simulink model "Assignement_Simulink"  (R2022b)
settings: Solver=ode8  StartTime=0.0  StopTime=50000  FixedStep=0.1  RelTol=1e-3
values from neighbouring files (symbols this model uses):
  a = 16371e3    (= 16371000)    [Assignement_Script.m]
  A0 = eye(3,3)    [Assignement_Script.m]
  A1 = 0.02    [Assignement_Script.m]
  A2 = A1    (= 0.02)    [Assignement_Script.m]
  A3 = A1    (= 0.02)    [Assignement_Script.m]
  alpha_1 = 0.5    [Assignement_Script.m]
  alpha_2 = 0.5    [Assignement_Script.m]
  C_d = 2.1    [Assignement_Script.m]
  e = 0    [Assignement_Script.m]
  epsilon = 0.4093    [Assignement_Script.m]
  G = 6.6743e-11    [Assignement_Script.m]
  H0 = sqrt(g_10^2+g_11^2+h_11^2)    [Assignement_Script.m]
  i = 0.1    [Assignement_Script.m]
  I = 12/23.342 *diag([0.343,0.344,0.286])    [Assignement_Script.m]
  j_B = [0.01;0.05;0.01]    [Assignement_Script.m]
  k_d_detumbling = 0.12    [Assignement_Script.m]
  k_d_nadir = 0.12    [Assignement_Script.m]
  k_p_nadir = 0.12    [Assignement_Script.m]
  M_Earth = 5.972e24    (= 5.972e+24)    [Assignement_Script.m]
  n = sqrt(G*M_Earth/a^3)    [Assignement_Script.m]
  n_sun = 2*pi/T_sun    (= 1.99238499086e-07)    [Assignement_Script.m]
  omega_detumbling = [0; 0; n_SC]    [Assignement_Script.m]
  omega_nadir = omega_detumbling    [Assignement_Script.m]
  P = F_e/c    (= 4.52666666667e-06)    [Assignement_Script.m]
  position = 1e-2*[15,0,0;0,5,0;-15,0,0;0,-5,0;0,0,10;                                     0,0,-10;0,20,10;0,20,10;0,-20,10;0,-20,10]    [Assignement_Script.m]
  R_Earth = 6.378e6    (= 6378000)    [Assignement_Script.m]
  R_sun = 149597870000    [Assignement_Script.m]
  rhoD_vector = ones(10,1)*0.1    [Assignement_Script.m]
  rhoS_vector = ones(10,1)*0.5    [Assignement_Script.m]
  Surfaces_Matrix = [2e-2;6e-2;2e-2;6e-2;3e-2;3e-2;12e-2;                                                     12e-2;12e-2;12e-2]    [Assignement_Script.m]
  theta0 = 3/2*pi    (= 4.71238898038)    [Assignement_Script.m]
  Theta_m = deg2rad(11.5)    [Assignement_Script.m]
  time_detumbling = 500    [Assignement_Script.m]
  Versor_Surfaces_Matrix = [  1 , 0 ,-1 , 0 , 0 , 0 , 0 , 0 , 0 , 0 ... (first row only)    [Assignement_Script.m]
  w0 = [0;0;0.01]    [Assignement_Script.m]
  w_Earth = 7.2916e-5    (= 7.2916e-05)    [Assignement_Script.m]
undefined symbols (not defined in the file or in its folder): Gyroscope, HS, RW, SunSensor
libraries: simulink_extras x14, vrlib x11, matrix_library x10, sharedutil x10
(part 1 of 2)
settings Model: Creator=ludov  LastModifiedBy=ludov

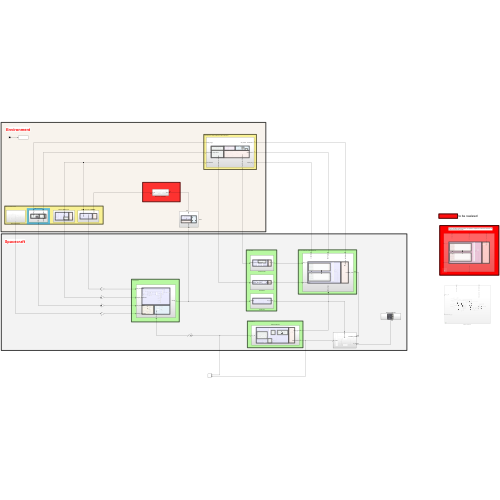
[thumbnail: Simulink's stored preview of the top-level diagram]
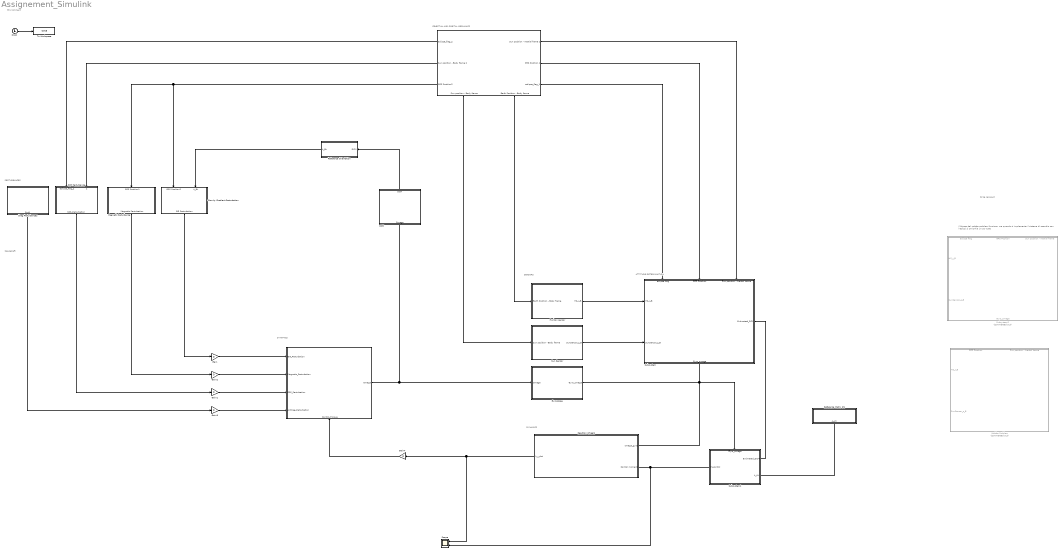
== system Assignement_Simulink ==
  note: il blocco del wabba problem funziona, ma quando si implementa il sistema di scambio con l'eclissi si smicnhia un po' tutto
  note: Environment
  note: ATTITUDE DETERMINATION
  note: to be rewiewd
  note: DYNAMICS
  note: SENSORS
  note: CELESTIAL AND ORBITAL MECHANICS
  note: PERTURBANCES
  note: Spacecraft
  note: DYNAMICS
  " " : Subsystem
      settings: PortSchema="{\"entries\":[{\"content\":{\"sides\":[{\"content\":{\"connectorIds\":[\"Out6\",\"Out7\",\"Out8\"]},\"type\":\"ConnectorPlacement.EquallySpacedRectSide\",\"uuid\":\"e47ba2f2-6418-4f5c-a13b-aa90bdbafa09\"},{\"content\":{\"connectorIds\":[\"Out1\",\"Out2\",\"Out3\"],\"side\":\"RIGHT\"},\"type\":\"ConnectorPlacement.EquallySpacedRectSide\",\"uuid\":\"03bc7c76-661c-4c4e-84cf-6f77fb49d6cb\"},{\"content\":{\"connectorIds\":[],\"side\":\"TOP\"},\"type\":\"ConnectorPlacement.EquallySpacedRectSide\",\"uuid\":\"b7f23859-8b5f-4f36-86dd-1ae14c2fa2a2\"},{\"content\":{\"connectorIds\":[\"Out4\",\"Out5\"],\"side\":\"BOTTOM\"},\"type\":\"ConnectorPlacement.EquallySpacedRectSide\",\"uuid\":\"86089f92-8549-4212-b188-d7aa2d93da25\"}]},\"type\":\"ConnectorPlacement.EquallySpacedConnector\",\"uuid\":\"9d05c9f0-b3f6-416c-9c64-67f4b43926de\"}],\"packageUris\":[\"http://schema.mathworks.com/mf0/Connector/R2020b\"],\"version\":\"1.0\"}"
  "  " : Subsystem
      settings: PortSchema="{\"entries\":[{\"content\":{\"sides\":[{\"content\":{\"connectorIds\":[\"In1\",\"In2\",\"In3\",\"In4\"]},\"type\":\"ConnectorPlacement.EquallySpacedRectSide\",\"uuid\":\"aab80584-571d-4a71-b544-a0aeb6cc6c33\"},{\"content\":{\"connectorIds\":[\"Out1\"],\"side\":\"RIGHT\"},\"type\":\"ConnectorPlacement.EquallySpacedRectSide\",\"uuid\":\"24834e7f-96cf-4bd4-9d1e-2a40a9329077\"},{\"content\":{\"connectorIds\":[],\"side\":\"TOP\"},\"type\":\"ConnectorPlacement.EquallySpacedRectSide\",\"uuid\":\"d2051258-9c4b-4932-9464-9f9a506b88fb\"},{\"content\":{\"connectorIds\":[\"In5\"],\"side\":\"BOTTOM\"},\"type\":\"ConnectorPlacement.EquallySpacedRectSide\",\"uuid\":\"d87f08de-6428-4147-8fa3-4a4fdf5058ef\"}]},\"type\":\"ConnectorPlacement.EquallySpacedConnector\",\"uuid\":\"040bda51-1336-4023-88c4-8bbc78e4cc03\"}],\"packageUris\":[\"http://schema.mathworks.com/mf0/Connector/R2020b\"],\"version\":\"1.0\"}"
  " Magnetic Perturbance " : Subsystem
      settings: PortSchema="{\"entries\":[{\"content\":{\"sides\":[{\"content\":{\"connectorIds\":[]},\"type\":\"ConnectorPlacement.EquallySpacedRectSide\",\"uuid\":\"f02812cb-12c0-4612-9b94-50dc5ff6800f\"},{\"content\":{\"connectorIds\":[],\"side\":\"RIGHT\"},\"type\":\"ConnectorPlacement.EquallySpacedRectSide\",\"uuid\":\"f399267d-7809-425c-9d5e-8a09b98f84d1\"},{\"content\":{\"connectorIds\":[\"In1\"],\"side\":\"TOP\"},\"type\":\"ConnectorPlacement.EquallySpacedRectSide\",\"uuid\":\"723c78fa-3a63-413c-a07c-383f30094b4e\"},{\"content\":{\"connectorIds\":[\"Out1\"],\"side\":\"BOTTOM\"},\"type\":\"ConnectorPlacement.EquallySpacedRectSide\",\"uuid\":\"6e581abe-40d1-4528-bc1e-881c860c6457\"}]},\"type\":\"ConnectorPlacement.EquallySpacedConnector\",\"uuid\":\"57020123-0faa-4eee-b688-9329c8cd004b\"}],\"packageUris\":[\"http://schema.mathworks.com/mf0/Connector/R2020b\"],\"version\":\"1.0\"}"
  " SRP Perturbance" : Subsystem
      settings: PortSchema="{\"entries\":[{\"content\":{\"sides\":[{\"content\":{\"connectorIds\":[]},\"type\":\"ConnectorPlacement.EquallySpacedRectSide\",\"uuid\":\"e985e879-37b8-4f0c-a60b-74d5e4b5102c\"},{\"content\":{\"connectorIds\":[],\"side\":\"RIGHT\"},\"type\":\"ConnectorPlacement.EquallySpacedRectSide\",\"uuid\":\"1f0cb419-685e-4dd3-ab14-45869a41b9c2\"},{\"content\":{\"connectorIds\":[\"In1\",\"In2\"],\"side\":\"TOP\"},\"type\":\"ConnectorPlacement.EquallySpacedRectSide\",\"uuid\":\"f8cfa143-02f3-47d6-960d-90021c53ea82\"},{\"content\":{\"connectorIds\":[\"Out1\"],\"side\":\"BOTTOM\"},\"type\":\"ConnectorPlacement.EquallySpacedRectSide\",\"uuid\":\"2a12fd6d-c4b7-49e6-8cbf-522d896783f6\"}]},\"type\":\"ConnectorPlacement.EquallySpacedConnector\",\"uuid\":\"8752746d-e23a-4760-aab6-3f1c0a06bc69\"}],\"packageUris\":[\"http://schema.mathworks.com/mf0/Connector/R2020b\"],\"version\":\"1.0\"}"
  Clock : Clock
  DCM : Subsystem
      settings: PortSchema="{\"entries\":[{\"content\":{\"sides\":[{\"content\":{\"connectorIds\":[]},\"type\":\"ConnectorPlacement.EquallySpacedRectSide\",\"uuid\":\"36de77ec-8153-48fc-ae5a-ad0b0e2d3ce0\"},{\"content\":{\"connectorIds\":[],\"side\":\"RIGHT\"},\"type\":\"ConnectorPlacement.EquallySpacedRectSide\",\"uuid\":\"5bb36846-76d5-425c-bf3c-97c4283359fa\"},{\"content\":{\"connectorIds\":[\"Out1\"],\"side\":\"TOP\"},\"type\":\"ConnectorPlacement.EquallySpacedRectSide\",\"uuid\":\"8effcbf1-f39c-4e11-8297-2eedf506960c\"},{\"content\":{\"connectorIds\":[\"In1\"],\"side\":\"BOTTOM\"},\"type\":\"ConnectorPlacement.EquallySpacedRectSide\",\"uuid\":\"d53277ca-d1bd-4bb5-ab75-f8d5bccd248f\"}]},\"type\":\"ConnectorPlacement.EquallySpacedConnector\",\"uuid\":\"1130cf8d-ea10-4dfb-b209-46460bb57623\"}],\"packageUris\":[\"http://schema.mathworks.com/mf0/Connector/R2020b\"],\"version\":\"1.0\"}"
  Drag Perturbances : Subsystem
      settings: PortSchema="{\"entries\":[{\"content\":{\"sides\":[{\"content\":{\"connectorIds\":[]},\"type\":\"ConnectorPlacement.EquallySpacedRectSide\",\"uuid\":\"890f3e81-eae3-4d82-b131-a6b55e2e4e7e\"},{\"content\":{\"connectorIds\":[],\"side\":\"RIGHT\"},\"type\":\"ConnectorPlacement.EquallySpacedRectSide\",\"uuid\":\"fd77badb-3975-40f3-b2ef-8bc06b5f839c\"},{\"content\":{\"connectorIds\":[],\"side\":\"TOP\"},\"type\":\"ConnectorPlacement.EquallySpacedRectSide\",\"uuid\":\"74a13749-9f47-4ab9-b559-aa1ff3776051\"},{\"content\":{\"connectorIds\":[\"Out1\"],\"side\":\"BOTTOM\"},\"type\":\"ConnectorPlacement.EquallySpacedRectSide\",\"uuid\":\"ad5dbb3d-b795-4ab1-8885-dcb70df44dd7\"}]},\"type\":\"ConnectorPlacement.EquallySpacedConnector\",\"uuid\":\"adbac40e-e9e4-4933-ac77-075f4cd465ab\"}],\"packageUris\":[\"http://schema.mathworks.com/mf0/Connector/R2020b\"],\"version\":\"1.0\"}"
  Gain{,1..4} (5 alike) : Gain  Gain=0
  Gravity Gradient Perturbation : Subsystem
      settings: PortSchema="{\"entries\":[{\"content\":{\"sides\":[{\"content\":{\"connectorIds\":[]},\"type\":\"ConnectorPlacement.EquallySpacedRectSide\",\"uuid\":\"0f339a99-129b-4972-909e-aa08984290af\"},{\"content\":{\"connectorIds\":[],\"side\":\"RIGHT\"},\"type\":\"ConnectorPlacement.EquallySpacedRectSide\",\"uuid\":\"c349fcfc-19e0-4c37-99ec-428747fba93f\"},{\"content\":{\"connectorIds\":[\"In1\",\"In2\"],\"side\":\"TOP\"},\"type\":\"ConnectorPlacement.EquallySpacedRectSide\",\"uuid\":\"2ac505f4-7a46-421c-9759-99416a32691b\"},{\"content\":{\"connectorIds\":[\"Out1\"],\"side\":\"BOTTOM\"},\"type\":\"ConnectorPlacement.EquallySpacedRectSide\",\"uuid\":\"46063fda-cf86-410f-90fc-74dd4707f3ff\"}]},\"type\":\"ConnectorPlacement.EquallySpacedConnector\",\"uuid\":\"8656328d-f6ad-4baa-a1ea-e4d5445b99d9\"}],\"packageUris\":[\"http://schema.mathworks.com/mf0/Connector/R2020b\"],\"version\":\"1.0\"}"
  Gyroscope : Subsystem
  Horizon sensor : Subsystem
  Reaction Wheels : Subsystem
  Reference Matrix #1 : Subsystem
      settings: PortSchema="{\"entries\":[{\"content\":{\"sides\":[{\"content\":{\"connectorIds\":[]},\"type\":\"ConnectorPlacement.EquallySpacedRectSide\",\"uuid\":\"bcca36cf-8ac8-4df2-8c27-820de1fbb3ba\"},{\"content\":{\"connectorIds\":[],\"side\":\"RIGHT\"},\"type\":\"ConnectorPlacement.EquallySpacedRectSide\",\"uuid\":\"8624ce1f-10a4-46ad-9e5b-1a912f6d00ca\"},{\"content\":{\"connectorIds\":[],\"side\":\"TOP\"},\"type\":\"ConnectorPlacement.EquallySpacedRectSide\",\"uuid\":\"93036ba9-ac54-41ed-8cce-c13b1508dd7a\"},{\"content\":{\"connectorIds\":[\"Out1\"],\"side\":\"BOTTOM\"},\"type\":\"ConnectorPlacement.EquallySpacedRectSide\",\"uuid\":\"73593883-c463-4775-a781-721666040d63\"}]},\"type\":\"ConnectorPlacement.EquallySpacedConnector\",\"uuid\":\"7208a640-a625-4ee7-a86a-82274cfadb5b\"}],\"packageUris\":[\"http://schema.mathworks.com/mf0/Connector/R2020b\"],\"version\":\"1.0\"}"
  Reference Orientation : Subsystem
  Scope : Scope  NumInputPorts=2
  Subsystem : Subsystem
      settings: PortSchema="{\"entries\":[{\"content\":{\"sides\":[{\"content\":{\"connectorIds\":[\"In1\",\"In2\"]},\"type\":\"ConnectorPlacement.EquallySpacedRectSide\",\"uuid\":\"904c8655-8bda-40bc-8851-83b785dfa15e\"},{\"content\":{\"connectorIds\":[\"Out1\"],\"side\":\"RIGHT\"},\"type\":\"ConnectorPlacement.EquallySpacedRectSide\",\"uuid\":\"2c7420fa-7058-46da-8085-0ee08a188acb\"},{\"content\":{\"connectorIds\":[\"In3\",\"In4\",\"In5\"],\"side\":\"TOP\"},\"type\":\"ConnectorPlacement.EquallySpacedRectSide\",\"uuid\":\"499ed007-25d9-4559-b35a-ae71d71143f6\"},{\"content\":{\"connectorIds\":[\"In6\"],\"side\":\"BOTTOM\"},\"type\":\"ConnectorPlacement.EquallySpacedRectSide\",\"uuid\":\"c0208a51-188e-4d0b-a2a2-f21f47979d66\"}]},\"type\":\"ConnectorPlacement.EquallySpacedConnector\",\"uuid\":\"16926250-8c74-4bf5-939a-452d45825930\"}],\"packageUris\":[\"http://schema.mathworks.com/mf0/Connector/R2020b\"],\"version\":\"1.0\"}"
  Subsystem1 : Subsystem
      settings: PortSchema="{\"entries\":[{\"content\":{\"sides\":[{\"content\":{\"connectorIds\":[\"In1\",\"In2\"]},\"type\":\"ConnectorPlacement.EquallySpacedRectSide\",\"uuid\":\"bcca36cf-8ac8-4df2-8c27-820de1fbb3ba\"},{\"content\":{\"connectorIds\":[\"Out1\"],\"side\":\"RIGHT\"},\"type\":\"ConnectorPlacement.EquallySpacedRectSide\",\"uuid\":\"8624ce1f-10a4-46ad-9e5b-1a912f6d00ca\"},{\"content\":{\"connectorIds\":[\"In3\"],\"side\":\"TOP\"},\"type\":\"ConnectorPlacement.EquallySpacedRectSide\",\"uuid\":\"93036ba9-ac54-41ed-8cce-c13b1508dd7a\"}]},\"type\":\"ConnectorPlacement.EquallySpacedConnector\",\"uuid\":\"7208a640-a625-4ee7-a86a-82274cfadb5b\"}],\"packageUris\":[\"http://schema.mathworks.com/mf0/Connector/R2020b\"],\"version\":\"1.0\"}"
  Subsystem2 : Subsystem  Commented=on
      settings: PortSchema="{\"entries\":[{\"content\":{\"sides\":[{\"content\":{\"connectorIds\":[\"In1\",\"In2\"]},\"type\":\"ConnectorPlacement.EquallySpacedRectSide\",\"uuid\":\"904c8655-8bda-40bc-8851-83b785dfa15e\"},{\"content\":{\"connectorIds\":[],\"side\":\"RIGHT\"},\"type\":\"ConnectorPlacement.EquallySpacedRectSide\",\"uuid\":\"2c7420fa-7058-46da-8085-0ee08a188acb\"},{\"content\":{\"connectorIds\":[\"In3\",\"In4\",\"In5\"],\"side\":\"TOP\"},\"type\":\"ConnectorPlacement.EquallySpacedRectSide\",\"uuid\":\"499ed007-25d9-4559-b35a-ae71d71143f6\"},{\"content\":{\"connectorIds\":[\"In6\"],\"side\":\"BOTTOM\"},\"type\":\"ConnectorPlacement.EquallySpacedRectSide\",\"uuid\":\"c0208a51-188e-4d0b-a2a2-f21f47979d66\"}]},\"type\":\"ConnectorPlacement.EquallySpacedConnector\",\"uuid\":\"16926250-8c74-4bf5-939a-452d45825930\"}],\"packageUris\":[\"http://schema.mathworks.com/mf0/Connector/R2020b\"],\"version\":\"1.0\"}"
  Sun Sensor : Subsystem
  To Workspace : ToWorkspace  VariableName=time  SampleTime=-1
  "Wabba Problem   " : Subsystem  Commented=on
      settings: PortSchema="{\"entries\":[{\"content\":{\"sides\":[{\"content\":{\"connectorIds\":[\"In1\",\"In2\"]},\"type\":\"ConnectorPlacement.EquallySpacedRectSide\",\"uuid\":\"692c6d3d-a8f2-499c-91a9-b0c93e98f75e\"},{\"content\":{\"connectorIds\":[],\"side\":\"RIGHT\"},\"type\":\"ConnectorPlacement.EquallySpacedRectSide\",\"uuid\":\"1ce742a3-ce52-440c-800e-89beb75c5b36\"},{\"content\":{\"connectorIds\":[\"In3\",\"In4\"],\"side\":\"TOP\"},\"type\":\"ConnectorPlacement.EquallySpacedRectSide\",\"uuid\":\"136b807f-193f-4c92-b740-36ee5afae013\"},{\"content\":{\"connectorIds\":[],\"side\":\"BOTTOM\"},\"type\":\"ConnectorPlacement.EquallySpacedRectSide\",\"uuid\":\"f63666af-b04e-4ebd-b890-e9da3a257b46\"}]},\"type\":\"ConnectorPlacement.EquallySpacedConnector\",\"uuid\":\"09b5b65f-bc7f-44eb-8e09-c61a35babfb4\"}],\"packageUris\":[\"http://schema.mathworks.com/mf0/Connector/R2020b\"],\"version\":\"1.0\"}"
  wires:
  DCM/1(DCM) -> Reference Orientation/1(DCM)
  "  "/1(Omega) -> DCM/1(Omega), Gyroscope/1(Omega)
  " SRP Perturbance"/1(SRP_Perturbation) -> Gain1/1
  " Magnetic Perturbance "/1(Magnetic Perturbation) -> Gain2/1
  Drag Perturbances/1(Out1) -> Gain3/1
  Reference Orientation/1(A_BL) -> Gravity Gradient Perturbation/2(A_BL)
  Gravity Gradient Perturbation/1(GG Perturbation) -> Gain/1
  " "/5(Earth Position - Body frame) -> Horizon sensor/1(Earth Position - Body frame)
  " "/4(Sun position - Body frame) -> Sun Sensor/1(Sun position - Body frame)
  " "/3(eclipse_flag_1) -> Subsystem/3(eclipse flag)
  " "/1(Sun position - Inertial frame 1) -> Subsystem/5(Sun position - Inertial frame)
  " "/2(GPS Position 1) -> Subsystem/4(GPS Position)
  Gain/1 -> "  "/1(GG_Perturbation)
  Gain1/1 -> "  "/3(SRP_Perturbation)
  Gain2/1 -> "  "/2(Magnetic_Perturbation)
  Gain3/1 -> "  "/4(AirDrag_Perturbation)
  Gyroscope/1(Gyro_omega) -> Reaction Wheels/1(omega_gyro), Subsystem1/3(Gyro_omega), Subsystem/6(Gyro_omega)
  Horizon sensor/1(HS_r_B) -> Subsystem/1(HS_r_B)
  Sun Sensor/1(SunSensor_s_B) -> Subsystem/2(SunSensor_s_B)
  " "/8(GPS Position2) -> " Magnetic Perturbance "/1(GPS Position1), Gravity Gradient Perturbation/1(GPS Position2)
  " "/7(Sun position - Body frame 2) -> " SRP Perturbance"/2(Sun position - Inertial frame 2)
  Reaction Wheels/1(h_r_dot) -> Scope/1, Gain4/1
  Clock/1 -> To Workspace/1
  " "/6(eclipse_flag_2) -> " SRP Perturbance"/1(eclipse_flag_2)
  Subsystem1/1(M_control) -> Scope/2, Reaction Wheels/2(Control moment)
  Gain4/1 -> "  "/5(Control_Torque)
  Reference Matrix #1/1(A_LN) -> Subsystem1/2(A_LN)
  Subsystem/1(Extimated_DCM) -> Subsystem1/1(Extimated_DCM)

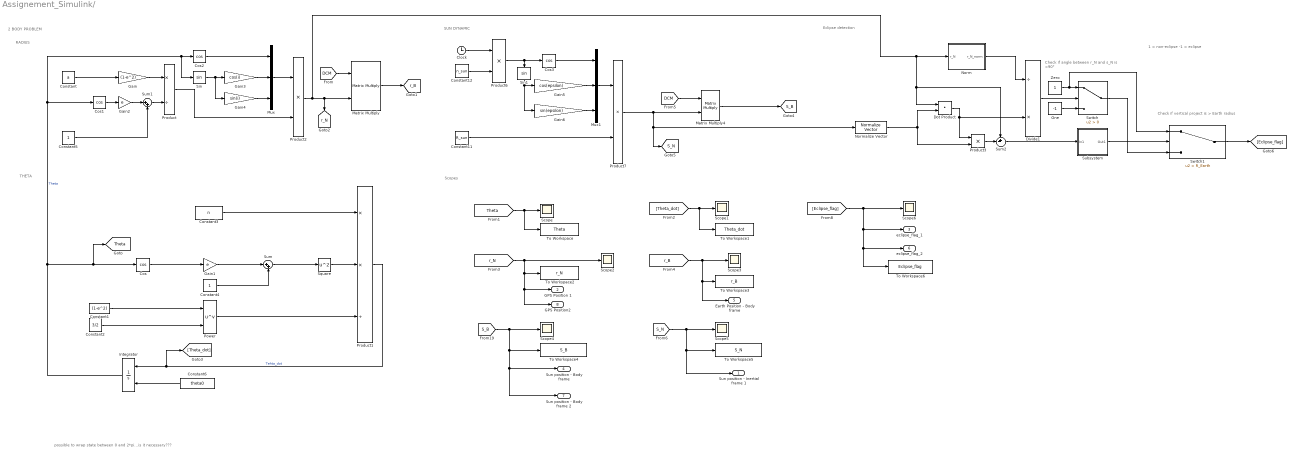
== system Assignement_Simulink/  ==
  note: 1 = non-eclipse
      | -1 = eclipse
  note: Check if vertical project is > Earth
      |  radius
  note: Check if angle between r_N
      |  and s_N is >90°
  note: Eclipse detection
  note: possible to wrap state between 0 and 2*pi...is it necessary???
  note: RADIUS
  note: 2 BODY PROBLEM
  note: THETA
  note: Scopes
  note: SUN DYNAMIC
  Clock : Clock
  Constant : Constant  Value=a
  Constant1 : Constant  Value=(1-e^2)
  Constant11 : Constant  Value=R_sun
  Constant12 : Constant  Value=n_sun
  Constant2 : Constant  Value=3/2
  Constant3 : Constant  Value=n
  Constant4 : Constant
  Constant5 : Constant
  Constant6 : Constant  Value=theta0
  Cos{,1..3} (4 alike) : Trigonometry  Operator=cos
  Divide1 : Product  Inputs=/*
  Dot Product : DotProduct  OutDataTypeStr=Inherit: Inherit via internal rule
  Gain : Gain  Gain=(1-e^2)
  Gain1 : Gain  Gain=e
  Gain2 : Gain  Gain=e
  Gain3 : Gain  Gain=cos(i)
  Gain4 : Gain  Gain=sin(i)
  Gain5 : Gain  Gain=cos(epsilon)
  Gain6 : Gain  Gain=sin(epsilon)
  Integrator : Integrator  InitialConditionSource=external  WrappedStateUpperValue=2*pi  WrappedStateLowerValue=0
  Matrix Multiply : Product  Multiplication=Matrix(*)
  Matrix Multiply4 : Product  Multiplication=Matrix(*)
  Mux : Mux  Inputs=3
  Mux1 : Mux  Inputs=3
  Norm : Subsystem
  Normalize Vector : vrlib/Utilities/Normalize Vector  maxzero=0
  One : Constant  Value=-1  OutDataTypeStr=Inherit: Inherit via back propagation
  Power : Math  Operator=pow
  Product : Product  Inputs=*/
  Product1 : Product  Inputs=**/
  Product{2..3,6..7} (4 alike) : Product
  Scope{,1..6} (7 alike) : Scope
  Sin : Trigonometry
  Sin1 : Trigonometry
  Square : Math  Operator=square
  Subsystem : Subsystem
  Sum : Sum  Inputs=|++
  Sum1 : Sum  Inputs=|++
  Sum2 : Sum  Inputs=+-|
  Switch : Switch  Criteria=u2 > Threshold  SaturateOnIntegerOverflow=off  InputSameDT=off
  Switch1 : Switch  Criteria=u2 > Threshold  Threshold=R_Earth  SaturateOnIntegerOverflow=off  InputSameDT=off
  To Workspace : ToWorkspace  VariableName=Theta  SampleTime=-1
  To Workspace1 : ToWorkspace  VariableName=Theta_dot  SampleTime=-1
  To Workspace2 : ToWorkspace  VariableName=r_N  SampleTime=-1
  To Workspace3 : ToWorkspace  VariableName=r_B  SampleTime=-1
  To Workspace4 : ToWorkspace  VariableName=S_B  SampleTime=-1
  To Workspace5 : ToWorkspace  VariableName=S_N  SampleTime=-1
  To Workspace6 : ToWorkspace  VariableName=Eclipse_flag  SampleTime=-1
  Zero : Constant  OutDataTypeStr=Inherit: Inherit via back propagation
  Sun position - Inertial frame 1 : Outport
  GPS Position 1 : Outport  Port=2
  eclipse_flag_1 : Outport  Port=3
  Sun position - Body frame : Outport  Port=4
  Earth Position - Body frame : Outport  Port=5
  eclipse_flag_2 : Outport  Port=6
  Sun position - Body frame 2 : Outport  Port=7
  GPS Position2 : Outport  Port=8
  tag scope: S_B=global, S_N=global, Theta=global, r_B=global, r_N=global
  wires:
  Constant/1 -> Gain/1
  Gain/1 -> Product/1
  Constant3/1 -> Product1/1
  Cos/1 -> Gain1/1
  Gain1/1 -> Sum/1
  Constant4/1 -> Sum/2
  Sum/1 -> Square/1
  Square/1 -> Product1/2
  Power/1 -> Product1/3
  Constant1/1 -> Power/1
  Constant2/1 -> Power/2
  Product1/1 -> [Theta_dot], Integrator/1  "Tehta_dot"
  Integrator/1 -> Cos2/1, Sin/1, Cos1/1, [Theta], Cos/1  "Theta"
  Cos1/1 -> Gain2/1
  Constant5/1 -> Sum1/2
  Gain2/1 -> Sum1/1
  Sum1/1 -> Product/2
  Constant6/1 -> Integrator/2
  Cos2/1 -> Mux/1
  Sin/1 -> Gain3/1, Gain4/1
  Gain3/1 -> Mux/2
  Gain4/1 -> Mux/3
  Mux/1 -> Product2/1
  Product/1 -> Product2/2
  Matrix Multiply/1 -> [r_B]
  [DCM] -> Matrix Multiply/1
  [Theta_dot] -> To Workspace1/1, Scope1/1
  [Theta] -> To Workspace/1, Scope/1
  Clock/1 -> Product6/1
  Sin1/1 -> Gain6/1, Gain5/1
  Constant11/1 -> Product7/2
  Mux1/1 -> Product7/1
  Product6/1 -> Sin1/1, Cos3/1
  Cos3/1 -> Mux1/1
  Constant12/1 -> Product6/2
  Gain6/1 -> Mux1/3
  Gain5/1 -> Mux1/2
  [DCM] -> Matrix Multiply4/1
  [S_B] -> Scope4/1, Sun position - Body frame 2/1, Sun position - Body frame/1, To Workspace4/1
  [r_B] -> Scope3/1, To Workspace3/1, Earth Position - Body frame/1
  [S_N] -> Sun position - Inertial frame 1/1, To Workspace5/1, Scope5/1
  Divide1/1 -> Switch/2
  Switch/1 -> Switch1/3
  Dot Product/1 -> Product3/1, Divide1/2
  Product7/1 -> Matrix Multiply4/2, [S_N], Normalize Vector/1
  Product2/1 -> Matrix Multiply/2, [r_N], Sum2/1, Dot Product/1, Norm/1(r_N)
  One/1 -> Switch/3
  Normalize Vector/1 -> Dot Product/2, Product3/2
  Product3/1 -> Sum2/2
  Zero/1 -> Switch1/1, Switch/1
  Norm/1(r_N_norm) -> Divide1/1
  Sum2/1 -> Subsystem/1(In1)
  Subsystem/1(Out1) -> Switch1/2
  Matrix Multiply4/1 -> [S_B]
  [r_N] -> Scope2/1, GPS Position2/1, GPS Position 1/1, To Workspace2/1
  Switch1/1 -> [Eclipse_flag]
  [Eclipse_flag] -> eclipse_flag_1/1, To Workspace6/1, eclipse_flag_2/1, Scope6/1

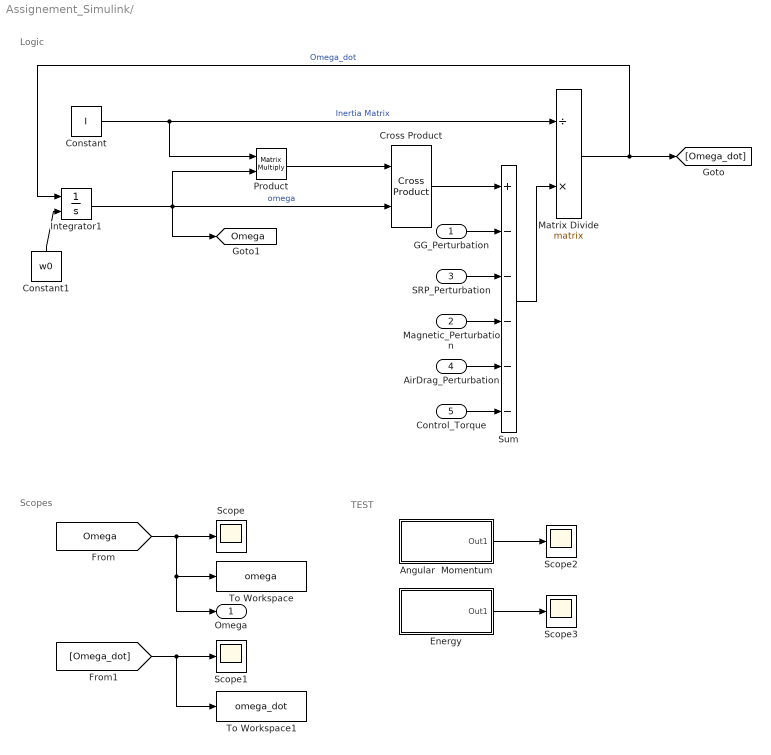
== system Assignement_Simulink/   ==
  note: TEST
  note: Logic
  note: Scopes
  GG_Perturbation : Inport
  Magnetic_Perturbation : Inport  Port=2
  SRP_Perturbation : Inport  Port=3
  AirDrag_Perturbation : Inport  Port=4
  Control_Torque : Inport  Port=5
  Angular  Momentum : Subsystem
  Constant : Constant  Value=I
  Constant1 : Constant  Value=w0
  Cross Product : matrix_library/Cross Product
  Energy : Subsystem
  Integrator1 : Integrator  InitialConditionSource=external  InitialCondition=w0
  Matrix Divide : Product  Inputs=/*  Multiplication=Matrix(*)
  Product : Product  Multiplication=Matrix(*)
  Scope{,1..3} (4 alike) : Scope
  Sum : Sum  Inputs=+-----
  To Workspace : ToWorkspace  VariableName=omega  SaveFormat=Timeseries  SampleTime=-1
  To Workspace1 : ToWorkspace  VariableName=omega_dot  SaveFormat=Timeseries  SampleTime=-1
  Omega : Outport
  tag scope: Omega=global
  wires:
  Product/1 -> Cross Product/1
  Integrator1/1 -> Cross Product/2, Product/2, [Omega]  "omega"
  Matrix Divide/1 -> [Omega_dot], Integrator1/1  "Omega_dot"
  Constant/1 -> Product/1, Matrix Divide/1  "Inertia Matrix"
  [Omega] -> Omega/1, To Workspace/1, Scope/1
  [Omega_dot] -> To Workspace1/1, Scope1/1
  Angular  Momentum/1(Out1) -> Scope2/1
  Energy/1(Out1) -> Scope3/1
  Constant1/1 -> Integrator1/2
  Cross Product/1 -> Sum/1
  Sum/1 -> Matrix Divide/2
  GG_Perturbation/1 -> Sum/2
  Magnetic_Perturbation/1 -> Sum/4
  SRP_Perturbation/1 -> Sum/3
  AirDrag_Perturbation/1 -> Sum/5
  Control_Torque/1 -> Sum/6

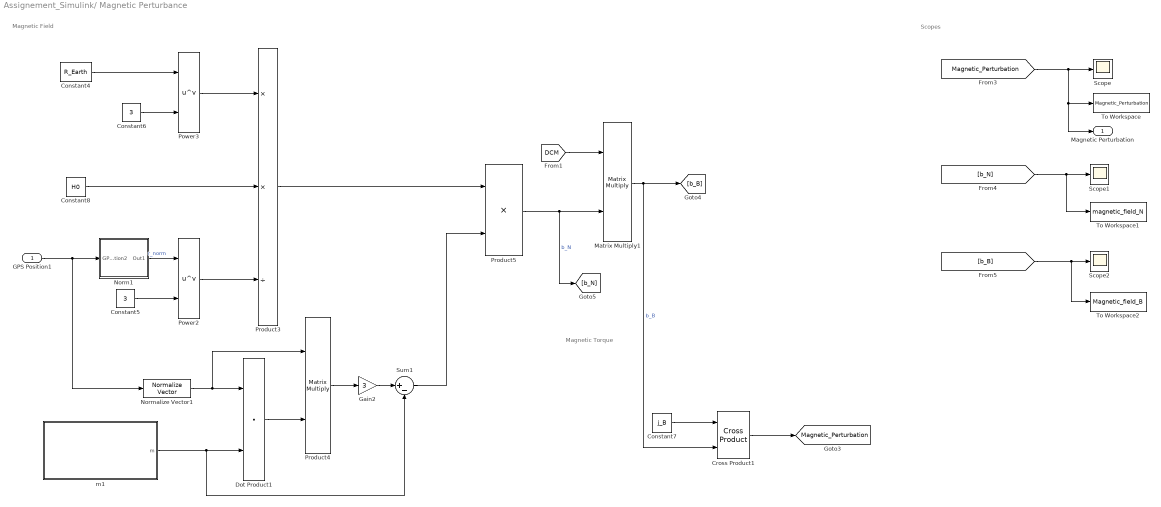
== system Assignement_Simulink/ Magnetic Perturbance  ==
  note: Scopes
  note: Magnetic Torque
  note: Magnetic Field
  GPS Position1 : Inport
  Constant4 : Constant  Value=R_Earth
  Constant5 : Constant  Value=3
  Constant6 : Constant  Value=3
  Constant7 : Constant  Value=j_B
  Constant8 : Constant  Value=H0
  Cross Product1 : matrix_library/Cross Product
  Dot Product1 : DotProduct  OutDataTypeStr=Inherit: Inherit via internal rule
  Gain2 : Gain  Gain=3
  Matrix Multiply1 : Product  Multiplication=Matrix(*)
  Norm1 : Subsystem
  Normalize Vector1 : vrlib/Utilities/Normalize Vector  maxzero=0
  Power2 : Math  Operator=pow
  Power3 : Math  Operator=pow
  Product3 : Product  Inputs=**/
  Product4 : Product  Multiplication=Matrix(*)
  Product5 : Product
  Scope : Scope
  Scope1 : Scope
  Scope2 : Scope
  Sum1 : Sum  Inputs=|+-
  To Workspace : ToWorkspace  VariableName=Magnetic_Perturbation  SampleTime=-1
  To Workspace1 : ToWorkspace  VariableName=magnetic_field_N  SaveFormat=Timeseries  SampleTime=-1
  To Workspace2 : ToWorkspace  VariableName=Magnetic_field_B  SaveFormat=Timeseries  SampleTime=-1
  m1 : Subsystem
  Magnetic Perturbation : Outport
  tag scope: Magnetic_Perturbation=global
  wires:
  [Magnetic_Perturbation] -> Scope/1, Magnetic Perturbation/1, To Workspace/1
  [b_N] -> To Workspace1/1, Scope1/1
  [b_B] -> To Workspace2/1, Scope2/1
  Product5/1 -> [b_N], Matrix Multiply1/2  "b_N"
  Constant8/1 -> Product3/2
  Matrix Multiply1/1 -> [b_B], Cross Product1/2  "b_B"
  Constant7/1 -> Cross Product1/1
  m1/1(m) -> Sum1/2, Dot Product1/2
  Product3/1 -> Product5/1
  Product4/1 -> Gain2/1
  Dot Product1/1 -> Product4/2
  Gain2/1 -> Sum1/1
  Cross Product1/1 -> [Magnetic_Perturbation]
  Normalize Vector1/1 -> Product4/1, Dot Product1/1
  Norm1/1(Out1) -> Power2/1  "r_norm"
  Sum1/1 -> Product5/2
  Power2/1 -> Product3/3
  Power3/1 -> Product3/1
  Constant6/1 -> Power3/2
  Constant5/1 -> Power2/2
  GPS Position1/1 -> Normalize Vector1/1, Norm1/1(GPS Position2)
  Constant4/1 -> Power3/1
  [DCM] -> Matrix Multiply1/1

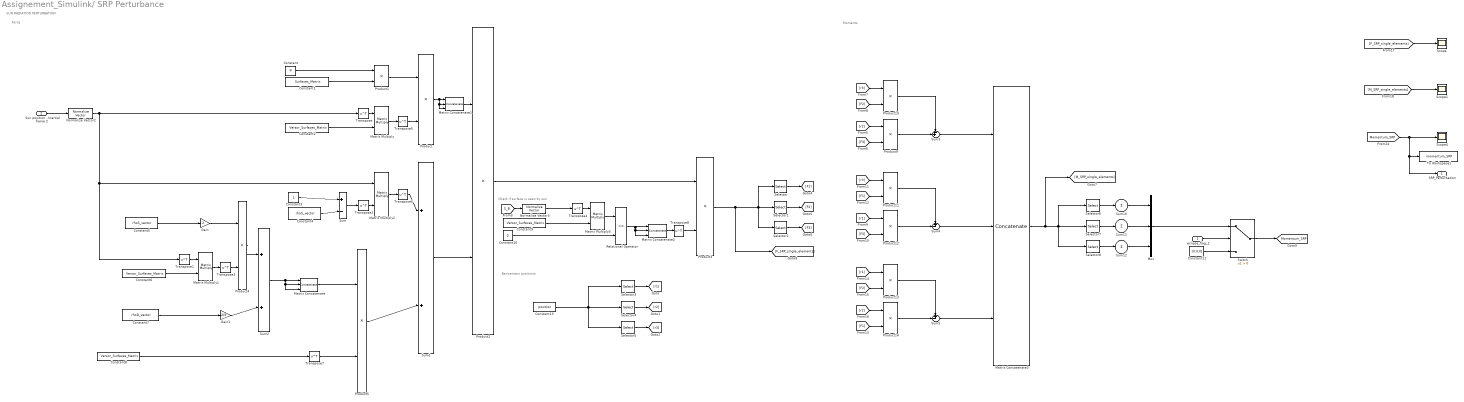
== system Assignement_Simulink/ SRP Perturbance ==
  note: Moments
  note: Force
  note: Check if surface is seen by sun
  note: SUN RADIATION PERTURBATION
  note: Baricenters positions
  eclipse_flag_2 : Inport
  Sun position - Inertial frame 2 : Inport  Port=2
  Constant : Constant  Value=-P
  Constant1 : Constant  Value=Surfaces_Matrix
  Constant10 : Constant  Value=0
  Constant11 : Constant  Value=[0;0;0]
  Constant13 : Constant  Value=position
  Constant{2,6,8..9} (4 alike) : Constant  Value=Versor_Surfaces_Matrix
  Constant3 : Constant
  Constant4 : Constant  Value=rhoS_vector
  Constant5 : Constant  Value=rhoS_vector
  Constant7 : Constant  Value=rhoD_vector
  Gain : Gain  Gain=2
  Gain1 : Gain  Gain=2/3
  Matrix Concatenate : Concatenate  NumInputs=3  Mode=Multidimensional array  ConcatenateDimension=2
  Matrix Concatenate1 : Concatenate  NumInputs=3  Mode=Multidimensional array  ConcatenateDimension=2
  Matrix Concatenate2 : Concatenate  NumInputs=3  Mode=Multidimensional array
  Matrix Concatenate3 : Concatenate  NumInputs=3  Mode=Multidimensional array  ConcatenateDimension=2
  Matrix Multiply{,1..3} (4 alike) : Product  Multiplication=Matrix(*)
  Mux : Mux  Inputs=3
  Normalize Vector2 : vrlib/Utilities/Normalize Vector  maxzero=0
  Normalize Vector3 : vrlib/Utilities/Normalize Vector  maxzero=0
  Product{,1..5,9..14} (12 alike) : Product
  Relational Operator : RelationalOperator  OutDataTypeStr=boolean  RndMeth=Simplest  InputSameDT=off
  Scope : Scope
  Scope1 : Scope
  Scope4 : Scope
  Selector : Selector  NumberOfDimensions=2  InputPortWidth=3  IndexOptions=Select all,Index vector (dialog)  Indices=1,1  OutputSizes=1,1
  Selector1 : Selector  NumberOfDimensions=2  InputPortWidth=3  IndexOptions=Select all,Index vector (dialog)  Indices=1,2  OutputSizes=1,1
  Selector2 : Selector  NumberOfDimensions=2  InputPortWidth=3  IndexOptions=Select all,Index vector (dialog)  Indices=1,3  OutputSizes=1,1
  Selector3 : Selector  NumberOfDimensions=2  InputPortWidth=3  IndexOptions=Select all,Index vector (dialog)  Indices=1,1  OutputSizes=1,1
  Selector4 : Selector  NumberOfDimensions=2  InputPortWidth=3  IndexOptions=Select all,Index vector (dialog)  Indices=1,2  OutputSizes=1,1
  Selector5 : Selector  NumberOfDimensions=2  InputPortWidth=3  IndexOptions=Select all,Index vector (dialog)  Indices=1,3  OutputSizes=1,1
  Selector6 : Selector  NumberOfDimensions=2  InputPortWidth=3  IndexOptions=Select all,Index vector (dialog)  Indices=[1 3],1  OutputSizes=1,1
  Selector7 : Selector  NumberOfDimensions=2  InputPortWidth=3  IndexOptions=Select all,Index vector (dialog)  Indices=[1 3],2  OutputSizes=1,1
  Selector8 : Selector  NumberOfDimensions=2  InputPortWidth=3  IndexOptions=Select all,Index vector (dialog)  Indices=[1 3],3  OutputSizes=1,1
  Sum : Sum  Inputs=+|-
  Sum1 : Sum  Inputs=+|+
  Sum10 : Sum  Inputs=+
  Sum11 : Sum  Inputs=+
  Sum12 : Sum  Inputs=+
  Sum2 : Sum  Inputs=+|+
  Sum3 : Sum  Inputs=-+|
  Sum4 : Sum  Inputs=+-|
  Sum5 : Sum  Inputs=+-|
  Switch : Switch  Criteria=u2 > Threshold  SaturateOnIntegerOverflow=off  InputSameDT=off
  To Workspace1 : ToWorkspace  VariableName=momentum_SRP  SampleTime=-1
  Transpose{,1..8} (9 alike) : Math  Operator=transpose
  SRP_Perturbation : Outport
  tag scope: Momentum_SRP=global
  wires:
  Constant/1 -> Product1/1
  Product1/1 -> Product/1
  Constant1/1 -> Product1/2
  Matrix Multiply/1 -> Transpose5/1
  Sun position - Inertial frame 2/1 -> Normalize Vector2/1
  Constant2/1 -> Matrix Multiply/2
  Constant3/1 -> Sum/1
  Constant4/1 -> Sum/2
  Transpose/1 -> Matrix Multiply/1
  Constant5/1 -> Gain/1
  Constant6/1 -> Matrix Multiply1/2
  Matrix Multiply1/1 -> Transpose3/1
  Gain/1 -> Product4/1
  Constant7/1 -> Gain1/1
  Matrix Multiply2/1 -> Transpose6/1
  Sum/1 -> Transpose2/1
  Transpose2/1 -> Matrix Multiply2/2
  Gain1/1 -> Sum2/2
  Transpose5/1 -> Product/2
  Product4/1 -> Sum2/1
  Transpose1/1 -> Matrix Multiply1/1
  Transpose3/1 -> Product4/2
  Product5/1 -> Sum1/2
  Transpose6/1 -> Sum1/1
  Constant8/1 -> Transpose7/1
  Transpose7/1 -> Product5/2
  Sum2/1 -> Matrix Concatenate/3, Matrix Concatenate/2, Matrix Concatenate/1
  Matrix Concatenate/1 -> Product5/1
  Product/1 -> Matrix Concatenate1/3, Matrix Concatenate1/2, Matrix Concatenate1/1
  Matrix Concatenate1/1 -> Product2/1
  Constant10/1 -> Relational Operator/2
  Sum1/1 -> Product2/2
  [S_B] -> Normalize Vector3/1
  Matrix Multiply3/1 -> Relational Operator/1
  Transpose4/1 -> Matrix Multiply3/1
  Constant9/1 -> Matrix Multiply3/2
  Relational Operator/1 -> Matrix Concatenate2/3, Matrix Concatenate2/2, Matrix Concatenate2/1
  Matrix Concatenate2/1 -> Transpose8/1
  Product2/1 -> Product3/1
  Transpose8/1 -> Product3/2
  Product3/1 -> [F_SRP_single_elements], Selector/1, Selector2/1, Selector1/1
  Constant13/1 -> Selector5/1, Selector4/1, Selector3/1
  Selector3/1 -> [r1]
  Selector4/1 -> [r2]
  Selector5/1 -> [r3]
  Selector/1 -> [F1]
  Selector1/1 -> [F2]
  Selector2/1 -> [F3]
  [r2] -> Product9/1
  [F3] -> Product9/2
  Product9/1 -> Sum3/2
  [F2] -> Product10/2
  [r3] -> Product10/1
  Product10/1 -> Sum3/1
  Product12/1 -> Sum4/2
  [F3] -> Product12/2
  [r1] -> Product12/1
  [r3] -> Product11/1
  [F1] -> Product11/2
  Product11/1 -> Sum4/1
  Product14/1 -> Sum5/2
  [F1] -> Product14/2
  Product13/1 -> Sum5/1
  [r2] -> Product14/1
  [F2] -> Product13/2
  [r1] -> Product13/1
  Sum5/1 -> Matrix Concatenate3/3
  Sum4/1 -> Matrix Concatenate3/2
  Sum3/1 -> Matrix Concatenate3/1
  Matrix Concatenate3/1 -> Selector6/1, Selector7/1, Selector8/1, [M_SRP_single_elements]
  [F_SRP_single_elements] -> Scope/1
  [M_SRP_single_elements] -> Scope1/1
  [Momentum_SRP] -> SRP_Perturbation/1, To Workspace1/1, Scope4/1
  Selector6/1 -> Sum10/1
  Selector7/1 -> Sum11/1
  Selector8/1 -> Sum12/1
  Sum12/1 -> Mux/3
  Sum11/1 -> Mux/2
  Sum10/1 -> Mux/1
  Normalize Vector2/1 -> Transpose/1, Transpose1/1, Matrix Multiply2/1
  Normalize Vector3/1 -> Transpose4/1
  Mux/1 -> Switch/1
  eclipse_flag_2/1 -> Switch/2
  Switch/1 -> [Momentum_SRP]
  Constant11/1 -> Switch/3

== system Assignement_Simulink/DCM ==
  note: SCOPES
  note: LOGIC
  note: TEST
  Omega : Inport
  Anti-symmetric Matrix : Subsystem
  Constant1 : Constant  Value=A0
  Gain1 : Gain  Gain=-1
  Integrator2 : Integrator  InitialConditionSource=external
  Matrix Multiply1 : Product  Multiplication=Matrix(*)
  Matrix determinant : Subsystem
  Ortonormalizzation : Subsystem
  Perpendicularity : Subsystem
  Scope : Scope
  Scope1 : Scope
  Scope2 : Scope
  To Workspace : ToWorkspace  VariableName=DCM  SaveFormat=Structure With Time  SampleTime=-1
  DCM : Outport
  tag scope: DCM=global
  wires:
  [DCM] -> To Workspace/1, Scope/1
  Anti-symmetric Matrix/1("[w]^") -> Matrix Multiply1/1
  Integrator2/1 -> Ortonormalizzation/1(In1)
  Matrix Multiply1/1 -> Gain1/1
  Ortonormalizzation/1(Output) -> Perpendicularity/1(DCM), Matrix determinant/1(DCM), Matrix Multiply1/2, DCM/1, [DCM]
  Omega/1 -> Anti-symmetric Matrix/1(Omega)
  Gain1/1 -> Integrator2/1
  Constant1/1 -> Integrator2/2
  Matrix determinant/1(Determinant) -> Scope1/1
  Perpendicularity/1(Perpendicularity flag) -> Scope2/1

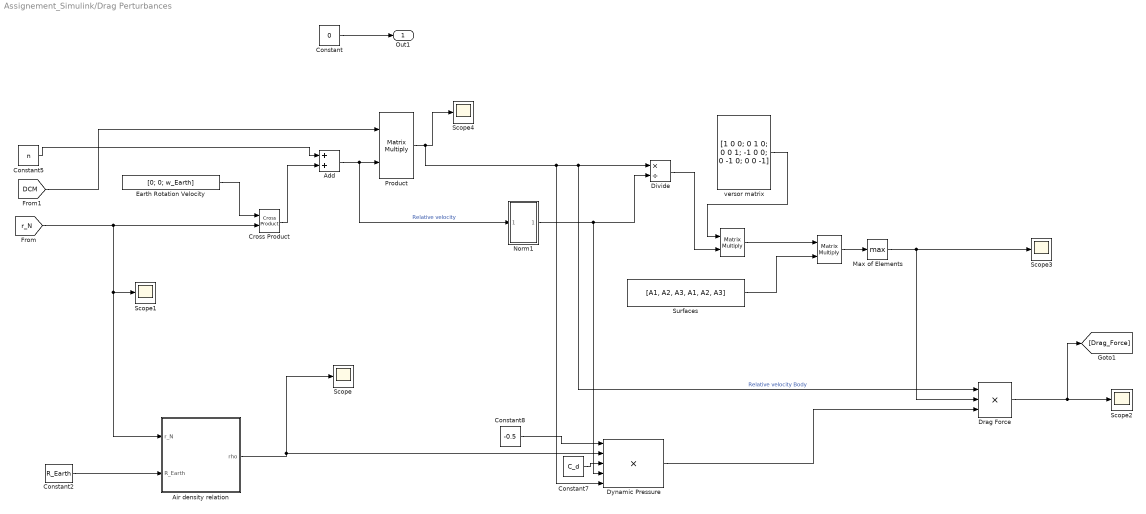
== system Assignement_Simulink/Drag Perturbances ==
  " " : Product  Multiplication=Matrix(*)
  "   " : Product  Multiplication=Matrix(*)
  Add : Sum
  Air density relation : MATLAB Function  TreatAsAtomicUnit=on
  Constant : Constant  Value=0
  Constant2 : Constant  Value=R_Earth
  Constant5 : Constant  Value=n
  Constant7 : Constant  Value=C_d
  Constant8 : Constant  Value=-0.5
  Cross Product : vrlib/Utilities/Cross Product
  Divide : Product  Inputs=*/
  Drag Force : Product  Inputs=***
  Dynamic Pressure : Product  Inputs=*****
  Earth Rotation Velocity : Constant  Value=[0; 0; w_Earth]
  Max of Elements : MinMax  Function=max
  Norm1 : Subsystem
  Product : Product  Multiplication=Matrix(*)
  Scope{,1..4} (5 alike) : Scope
  Surfaces : Constant  Value=[A1, A2, A3, A1, A2, A3]
  versor matrix : Constant  Value=[1 0 0; 0 1 0; 0 0 1; -1 0 0; 0 -1 0; 0 0 -1]
  Out1 : Outport
  wires:
  [DCM] -> Product/1
  [r_N] -> Scope1/1, Air density relation/1(r_N), Cross Product/2
  Drag Force/1 -> [Drag_Force], Scope2/1
  Constant8/1 -> Dynamic Pressure/1
  Cross Product/1 -> Add/2
  Add/1 -> Norm1/1(In1), Product/2  "Relative velocity"
  Product/1 -> Dynamic Pressure/5, Drag Force/1, Divide/1, Scope4/1  "Relative velocity Body"
  Norm1/1(Out1) -> Dynamic Pressure/4, Divide/2
  Air density relation/1(rho) -> Scope/1, Dynamic Pressure/2
  Earth Rotation Velocity/1 -> Cross Product/1
  Constant5/1 -> Add/1
  " "/1 -> Max of Elements/1
  Max of Elements/1 -> Drag Force/2, Scope3/1
  Dynamic Pressure/1 -> Drag Force/3
  Divide/1 -> "   "/2
  Surfaces/1 -> " "/2
  versor matrix/1 -> "   "/1
  Constant2/1 -> Air density relation/2(R_Earth)
  Constant7/1 -> Dynamic Pressure/3
  "   "/1 -> " "/1
  Constant/1 -> Out1/1

== system Assignement_Simulink/Gravity Gradient Perturbation ==
  note: Gravity Gradient Perturbation
  GPS Position2 : Inport
  A_BL : Inport  Port=2
  Constant : Constant  Value=[1;0;0]
  Constant1 : Constant  Value=3
  Constant3 : Constant  Value=I
  Cross Product2 : matrix_library/Cross Product
  Gain1 : Gain  Gain=3*G*M_Earth
  Matrix Multiply : Product  Multiplication=Matrix(*)
  Matrix Multiply1 : Product  Multiplication=Matrix(*)
  Norm : Subsystem
  Power : Math  Operator=pow
  Product : Product  Inputs=*/
  Scope : Scope
  To Workspace : ToWorkspace  VariableName=GG_perturbation  SampleTime=-1
  GG Perturbation : Outport
  tag scope: GG_Perturbation=global
  wires:
  Constant3/1 -> Matrix Multiply1/1  "Inertia Matrix"
  Matrix Multiply1/1 -> Cross Product2/1
  Cross Product2/1 -> Gain1/1
  [GG_Perturbation] -> Scope/1, GG Perturbation/1, To Workspace/1
  Matrix Multiply/1 -> Matrix Multiply1/2, Cross Product2/2
  A_BL/1 -> Matrix Multiply/1
  Constant/1 -> Matrix Multiply/2
  Gain1/1 -> Product/1
  GPS Position2/1 -> Norm/1(In1)
  Power/1 -> Product/2
  Product/1 -> [GG_Perturbation]
  Constant1/1 -> Power/2
  Norm/1(Out1) -> Power/1  "r_norm"

== system Assignement_Simulink/Gyroscope ==
  Omega : Inport
  Bias : Bias  Bias=Gyroscope.bias_gyro  SaturateOnIntegerOverflow=off
  Constant : Constant  Value=Gyroscope.A_epsilon
  Degrees to Radians : simulink_extras/Transformations/Degrees to Radians
  Gain : Gain  Gain=Gyroscope.Gain
  Matrix Multiply1 : Product  Multiplication=Matrix(*)
  Radians to Degrees : simulink_extras/Transformations/Radians to Degrees
  Scope : Scope
  Scope1 : Scope
  Sum : Sum  Inputs=|++
  White Noise : RandomNumber  Mean=Gyroscope.ARW_mean_value  Variance=0.0001  SampleTime=Gyroscope.sample_time
  Zero-Order Hold : ZeroOrderHold  SampleTime=-1
  Gyro_omega : Outport
  wires:
  Gain/1 -> Sum/1
  Sum/1 -> Bias/1
  Bias/1 -> Zero-Order Hold/1
  Zero-Order Hold/1 -> Degrees to Radians/1
  Radians to Degrees/1 -> Gain/1
  Matrix Multiply1/1 -> Radians to Degrees/1, Scope1/1
  Degrees to Radians/1 -> Scope/1, Gyro_omega/1
  Constant/1 -> Matrix Multiply1/1
  Omega/1 -> Matrix Multiply1/2
  White Noise/1 -> Sum/2

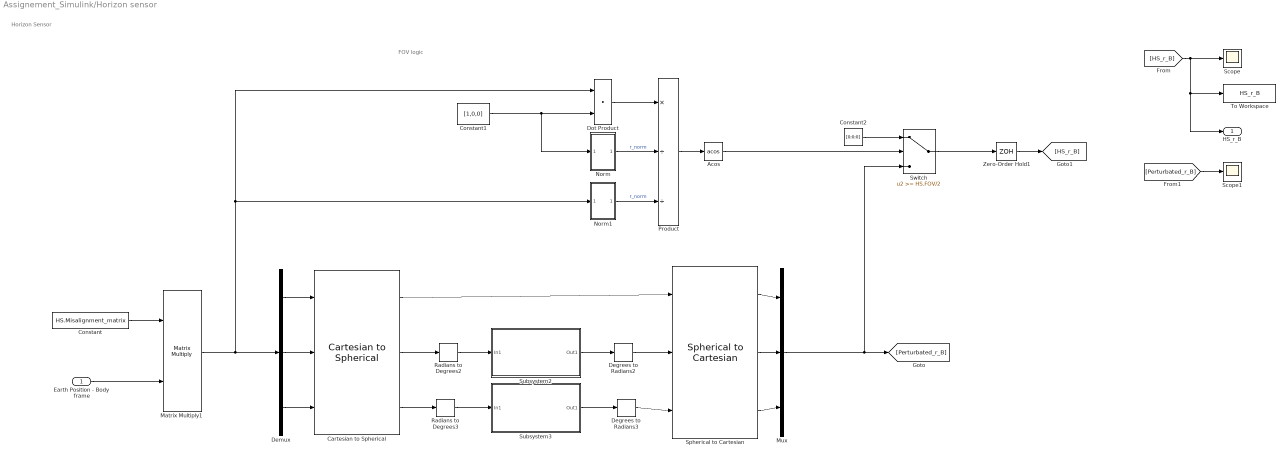
== system Assignement_Simulink/Horizon sensor ==
  note: Horizon Sensor
  note: FOV logic
  Earth Position - Body frame : Inport
  Acos : Trigonometry  Operator=acos
  Cartesian to Spherical : simulink_extras/Transformations/Cartesian to Spherical
  Constant : Constant  Value=HS.Misalignment_matrix
  Constant1 : Constant  Value=[1,0,0]
  Constant2 : Constant  Value=[0;0;0]
  Degrees to Radians2 : simulink_extras/Transformations/Degrees to Radians
  Degrees to Radians3 : simulink_extras/Transformations/Degrees to Radians
  Demux : Demux  Outputs=3
  Dot Product : DotProduct  OutDataTypeStr=Inherit: Inherit via internal rule
  Matrix Multiply1 : Product  Multiplication=Matrix(*)
  Mux : Mux  Inputs=3
  Norm : Subsystem
  Norm1 : Subsystem
  Product : Product  Inputs=*//
  Radians to Degrees2 : simulink_extras/Transformations/Radians to Degrees
  Radians to Degrees3 : simulink_extras/Transformations/Radians to Degrees
  Scope : Scope
  Scope1 : Scope
  Spherical to Cartesian : simulink_extras/Transformations/Spherical to Cartesian
  Subsystem2 : Subsystem
  Subsystem3 : Subsystem
  Switch : Switch  Threshold=HS.FOV/2  SaturateOnIntegerOverflow=off  InputSameDT=off
  To Workspace : ToWorkspace  VariableName=HS_r_B  SaveFormat=Timeseries  SampleTime=-1
  Zero-Order Hold1 : ZeroOrderHold  SampleTime=HS.sample_time
  HS_r_B : Outport
  wires:
  Constant/1 -> Matrix Multiply1/1
  Constant1/1 -> Dot Product/2, Norm/1(In1)
  Switch/1 -> Zero-Order Hold1/1
  Radians to Degrees3/1 -> Subsystem3/1(In1)
  Subsystem3/1(Out1) -> Degrees to Radians3/1
  Subsystem2/1(Out1) -> Degrees to Radians2/1
  Radians to Degrees2/1 -> Subsystem2/1(In1)
  Demux/1 -> Cartesian to Spherical/1
  Demux/2 -> Cartesian to Spherical/2
  Demux/3 -> Cartesian to Spherical/3
  Mux/1 -> [Perturbated_r_B], Switch/3
  Cartesian to Spherical/1 -> Spherical to Cartesian/1
  Spherical to Cartesian/3 -> Mux/3
  Spherical to Cartesian/2 -> Mux/2
  Spherical to Cartesian/1 -> Mux/1
  Cartesian to Spherical/2 -> Radians to Degrees2/1
  Degrees to Radians2/1 -> Spherical to Cartesian/2
  Cartesian to Spherical/3 -> Radians to Degrees3/1
  Degrees to Radians3/1 -> Spherical to Cartesian/3
  Matrix Multiply1/1 -> Dot Product/1, Norm1/1(In1), Demux/1
  Dot Product/1 -> Product/1
  Norm/1(Out1) -> Product/2  "r_norm"
  Norm1/1(Out1) -> Product/3  "r_norm"
  Product/1 -> Acos/1
  Acos/1 -> Switch/2
  Constant2/1 -> Switch/1
  Earth Position - Body frame/1 -> Matrix Multiply1/2
  Zero-Order Hold1/1 -> [HS_r_B]
  [HS_r_B] -> Scope/1, HS_r_B/1, To Workspace/1
  [Perturbated_r_B] -> Scope1/1

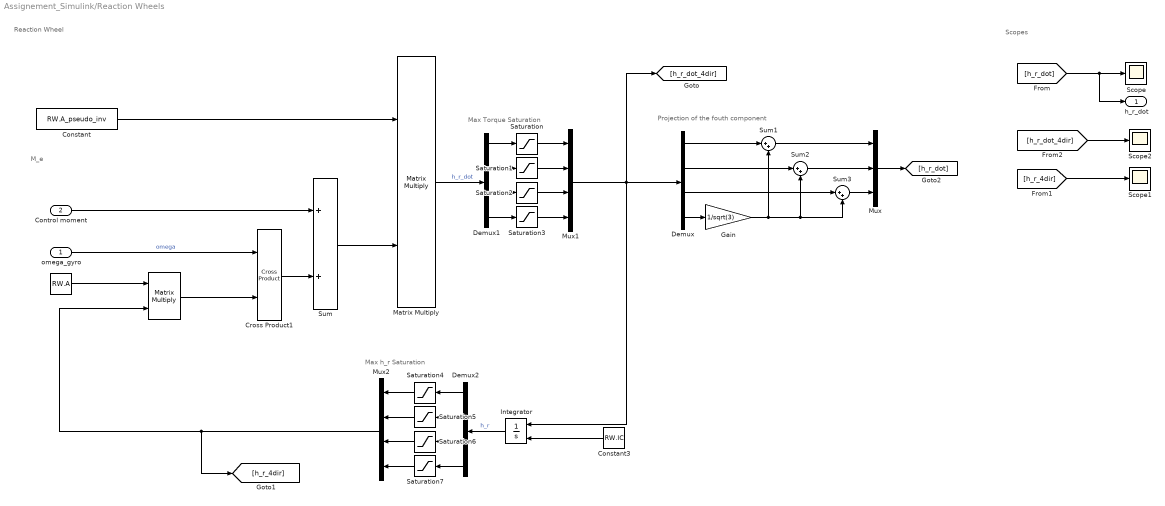
== system Assignement_Simulink/Reaction Wheels ==
  note: Max Torque Saturation
  note: Projection of the fouth component
  note: M_e
  note: Scopes
  note: Reaction Wheel
  note: Max h_r Saturation
  omega_gyro : Inport
  Control moment : Inport  Port=2
  " " : Constant  Value=RW.A
  "  " : Product  Multiplication=Matrix(*)
  Constant : Constant  Value=RW.A_pseudo_inv
  Constant3 : Constant  Value=RW.IC
  Cross Product1 : matrix_library/Cross Product
  Demux : Demux
  Demux1 : Demux
  Demux2 : Demux
  Gain : Gain  Gain=1/sqrt(3)
  Integrator : Integrator  InitialConditionSource=external
  Matrix Multiply : Product  Multiplication=Matrix(*)
  Mux : Mux  Inputs=3
  Mux1 : Mux
  Mux2 : Mux
  Saturation{,1..3} (4 alike) : Saturate  UpperLimit=RW.Max_torque_saturation  LowerLimit=-RW.Max_torque_saturation
  Saturation{4..7} (4 alike) : Saturate  UpperLimit=RW.Max_ang_mom_saturation  LowerLimit=-RW.Max_ang_mom_saturation
  Scope : Scope
  Scope1 : Scope
  Scope2 : Scope
  Sum : Sum
  Sum1 : Sum  Inputs=|++
  Sum2 : Sum  Inputs=|++
  Sum3 : Sum  Inputs=|++
  h_r_dot : Outport
  wires:
  Constant/1 -> Matrix Multiply/1
  Control moment/1 -> Sum/1
  Cross Product1/1 -> Sum/2
  " "/1 -> "  "/1
  omega_gyro/1 -> Cross Product1/1  "omega"
  "  "/1 -> Cross Product1/2
  Sum/1 -> Matrix Multiply/2
  Constant3/1 -> Integrator/2
  [h_r_dot] -> h_r_dot/1, Scope/1
  [h_r_4dir] -> Scope1/1
  Demux/1 -> Sum1/1
  Demux/2 -> Sum2/1
  Demux/3 -> Sum3/1
  Demux/4 -> Gain/1
  Gain/1 -> Sum3/2, Sum2/2, Sum1/2
  Sum1/1 -> Mux/1
  Sum2/1 -> Mux/2
  Sum3/1 -> Mux/3
  Integrator/1 -> Demux2/1  "h_r"
  Mux/1 -> [h_r_dot]
  [h_r_dot_4dir] -> Scope2/1
  Demux1/1 -> Saturation/1
  Mux1/1 -> Integrator/1, [h_r_dot_4dir], Demux/1
  Matrix Multiply/1 -> Demux1/1  "h_r_dot"
  Saturation/1 -> Mux1/1
  Saturation1/1 -> Mux1/2
  Demux1/2 -> Saturation1/1
  Saturation2/1 -> Mux1/3
  Demux1/3 -> Saturation2/1
  Saturation3/1 -> Mux1/4
  Demux1/4 -> Saturation3/1
  Demux2/2 -> Saturation5/1
  Demux2/4 -> Saturation7/1
  Saturation6/1 -> Mux2/3
  Saturation5/1 -> Mux2/2
  Demux2/3 -> Saturation6/1
  Saturation4/1 -> Mux2/1
  Demux2/1 -> Saturation4/1
  Saturation7/1 -> Mux2/4
  Mux2/1 -> "  "/2, [h_r_4dir]

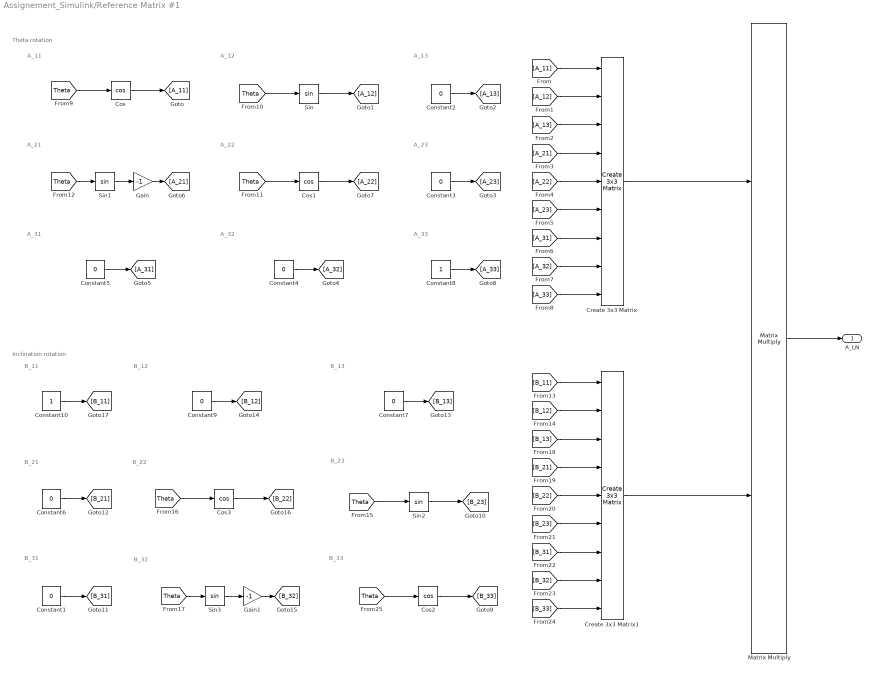
== system Assignement_Simulink/Reference Matrix #1 ==
  note: Theta rotation
  note: A_11
  note: A_12
  note: A_13
  note: A_23
  note: A_33
  note: A_22
  note: A_21
  note: A_31
  note: A_32
  note: B_22
  note: B_33
  note: B_13
  note: B_23
  note: Inclination rotation
  note: B_21
  note: B_32
  note: B_11
  note: B_31
  note: B_12
  Constant{1..7,9} (8 alike) : Constant  Value=0
  Constant10 : Constant
  Constant8 : Constant
  Cos{,1..3} (4 alike) : Trigonometry  Operator=cos
  Create 3x3 Matrix : sharedutil/Create 3x3 Matrix  aMode=aMode
      settings: LibrarySourceBlock=aerolibutil/Create 3x3 Matrix
  Create 3x3 Matrix1 : sharedutil/Create 3x3 Matrix  aMode=aMode
      settings: LibrarySourceBlock=aerolibutil/Create 3x3 Matrix
  Gain : Gain  Gain=-1
  Gain1 : Gain  Gain=-1
  Matrix Multiply : Product  Multiplication=Matrix(*)
  Sin{,1..3} (4 alike) : Trigonometry
  A_LN : Outport
  wires:
  [Theta] -> Cos/1
  Cos/1 -> [A_11]
  Sin/1 -> [A_12]
  Constant2/1 -> [A_13]
  Constant3/1 -> [A_23]
  Constant4/1 -> [A_32]
  Constant5/1 -> [A_31]
  Sin1/1 -> Gain/1
  Cos1/1 -> [A_22]
  Constant8/1 -> [A_33]
  [A_11] -> Create 3x3 Matrix/1
  [A_12] -> Create 3x3 Matrix/2
  [A_13] -> Create 3x3 Matrix/3
  [A_21] -> Create 3x3 Matrix/4
  [A_22] -> Create 3x3 Matrix/5
  [A_23] -> Create 3x3 Matrix/6
  [A_31] -> Create 3x3 Matrix/7
  [A_32] -> Create 3x3 Matrix/8
  [A_33] -> Create 3x3 Matrix/9
  Create 3x3 Matrix/1 -> Matrix Multiply/1
  [Theta] -> Sin/1
  [Theta] -> Cos1/1
  [Theta] -> Sin1/1
  Gain/1 -> [A_21]
  [Theta] -> Cos2/1
  [Theta] -> Sin3/1
  [Theta] -> Cos3/1
  [B_11] -> Create 3x3 Matrix1/1
  Constant6/1 -> [B_21]
  Constant10/1 -> [B_11]
  [B_12] -> Create 3x3 Matrix1/2
  Constant9/1 -> [B_12]
  Sin2/1 -> [B_23]
  Constant7/1 -> [B_13]
  Constant1/1 -> [B_31]
  Cos2/1 -> [B_33]
  Sin3/1 -> Gain1/1
  [B_23] -> Create 3x3 Matrix1/6
  [B_31] -> Create 3x3 Matrix1/7
  [B_33] -> Create 3x3 Matrix1/9
  Cos3/1 -> [B_22]
  Gain1/1 -> [B_32]
  [B_32] -> Create 3x3 Matrix1/8
  Create 3x3 Matrix1/1 -> Matrix Multiply/2
  [B_13] -> Create 3x3 Matrix1/3
  [Theta] -> Sin2/1
  [B_21] -> Create 3x3 Matrix1/4
  [B_22] -> Create 3x3 Matrix1/5
  Matrix Multiply/1 -> A_LN/1

== system Assignement_Simulink/Reference Orientation ==
  DCM : Inport
  Matrix Multiply : Product  Multiplication=Matrix(*)
  Reference Matrix #1 : Subsystem
  Scope : Scope
  To Workspace : ToWorkspace  VariableName=err  SampleTime=-1
  Transpose : Math  Operator=transpose
  A_BL : Outport
  wires:
  Transpose/1 -> Matrix Multiply/2
  Reference Matrix #1/1(A_LN) -> Transpose/1
  Matrix Multiply/1 -> Scope/1, To Workspace/1, A_BL/1
  DCM/1 -> Matrix Multiply/1

== system Assignement_Simulink/Subsystem ==
  note: Scopes
  HS_r_B : Inport
  SunSensor_s_B : Inport  Port=2
  eclipse flag : Inport  Port=3
  GPS Position : Inport  Port=4
  Sun position - Inertial frame : Inport  Port=5
  Gyro_omega : Inport  Port=6
  Algebraic method : Subsystem
  Bias : Bias  Bias=1  SaturateOnIntegerOverflow=off
  Delay : Delay  DelayLength=1
  Delay2 : Delay  DelayLength=1
  Gain : Gain  Gain=-1
  Gain1 : Gain  Gain=0.5
  Gyro propagation : Subsystem  TreatAsAtomicUnit=on
  Merge : Merge
  Scope : Scope
  To Workspace : ToWorkspace  VariableName=Extimated_DCM  SaveFormat=Timeseries  SampleTime=-1
  Extimated_DCM : Outport
  wires:
  Gyro_omega/1 -> Gyro propagation/2(Gyro_Omega)
  HS_r_B/1 -> Algebraic method/1(HS_r_B)
  SunSensor_s_B/1 -> Algebraic method/2(SunSensor_s_B)
  Sun position - Inertial frame/1 -> Algebraic method/3(Sun Position - Inerital frame)
  GPS Position/1 -> Algebraic method/4(GPS Position)
  Gyro propagation/1(Gyro_DCM) -> Merge/2
  Merge/1 -> Delay/1, [Extimated_DCM]
  Algebraic method/1(Calculated DCM) -> Merge/1
  Delay/1 -> Gyro propagation/3(Calculated DCM)  "Initial condition"
  [Extimated_DCM] -> Scope/1, Extimated_DCM/1, To Workspace/1
  eclipse flag/1 -> Gain/1, Algebraic method/Enable, Bias/1  "Initial condition"
  Gain/1 -> Gyro propagation/Enable
  Delay2/1 -> Gyro propagation/1(reset signal)
  Bias/1 -> Gain1/1
  Gain1/1 -> Delay2/1

== system Assignement_Simulink/Subsystem1 ==
  Extimated_DCM : Inport
  A_LN : Inport  Port=2
  Gyro_omega : Inport  Port=3
  Detumbling : Subsystem
  Nadir Pointing : Subsystem
  Sum : Sum  Inputs=|++
  Switch logic : Subsystem
  M_control : Outport
  wires:
  Switch logic/1(Detumbling) -> Detumbling/Enable
  Detumbling/1(M_detumbling) -> Sum/1
  Gyro_omega/1 -> Nadir Pointing/1(Gyro_omega), Detumbling/1(omega_gyro)
  Nadir Pointing/1(M_nadir) -> Sum/2
  Extimated_DCM/1 -> Nadir Pointing/2(Extimated_DCM)
  Switch logic/2(Nadir_pointing) -> Nadir Pointing/Enable
  Sum/1 -> M_control/1
  A_LN/1 -> Nadir Pointing/3(A_LN)

== system Assignement_Simulink/Subsystem2 ==
  note: Scopes
  HS_r_B : Inport
  SunSensor_s_B : Inport  Port=2
  eclipse flag : Inport  Port=3
  GPS Position : Inport  Port=4
  Sun position - Inertial frame : Inport  Port=5
  Gyro_omega : Inport  Port=6
  Algebraic method : Subsystem
  Bias : Bias  Bias=1  SaturateOnIntegerOverflow=off
  Delay : Delay  DelayLength=1
  Delay2 : Delay  DelayLength=1
  Gain : Gain  Gain=-1
  Gain1 : Gain  Gain=0.5
  Gyro propagation : Subsystem  TreatAsAtomicUnit=on
  Merge : Merge
  Scope : Scope
  wires:
  Gain1/1 -> Delay2/1
  Bias/1 -> Gain1/1
  Delay2/1 -> Gyro propagation/1(reset signal)
  Gain/1 -> Gyro propagation/Enable
  eclipse flag/1 -> Bias/1, Algebraic method/Enable, Gain/1  "Initial condition"
  [Extimated_DCM] -> Scope/1
  Delay/1 -> Gyro propagation/3(Calculated DCM)  "Initial condition"
  Algebraic method/1(Out1) -> Merge/1
  Merge/1 -> [Extimated_DCM], Delay/1
  Gyro propagation/1(Gyro_DCM) -> Merge/2
  GPS Position/1 -> Algebraic method/4(GPS Position)
  Sun position - Inertial frame/1 -> Algebraic method/3(Sun position - Inertial frame)
  SunSensor_s_B/1 -> Algebraic method/2(SunSensor_s_B)
  HS_r_B/1 -> Algebraic method/1(HS_r_B)
  Gyro_omega/1 -> Gyro propagation/2(Gyro_Omega)

== system Assignement_Simulink/Sun Sensor ==
  note: Scopes
  note: Horizon Sensor
  Sun position - Body frame : Inport
  Cartesian to Spherical : simulink_extras/Transformations/Cartesian to Spherical
  Constant : Constant  Value=SunSensor.Misalignment_matrix
  Degrees to Radians2 : simulink_extras/Transformations/Degrees to Radians
  Degrees to Radians3 : simulink_extras/Transformations/Degrees to Radians
  Demux : Demux  Outputs=3
  Matrix Multiply1 : Product  Multiplication=Matrix(*)
  Mux : Mux  Inputs=3
  Radians to Degrees2 : simulink_extras/Transformations/Radians to Degrees
  Radians to Degrees3 : simulink_extras/Transformations/Radians to Degrees
  Scope : Scope
  Spherical to Cartesian : simulink_extras/Transformations/Spherical to Cartesian
  Subsystem2 : Subsystem
  Subsystem3 : Subsystem
  To Workspace : ToWorkspace  VariableName=SunSensor_s_B  SaveFormat=Timeseries  SampleTime=-1
  Zero-Order Hold1 : ZeroOrderHold  SampleTime=HS.sample_time
  SunSensor_s_B : Outport
  wires:
  Constant/1 -> Matrix Multiply1/1
  Radians to Degrees3/1 -> Subsystem3/1(In1)
  Subsystem3/1(Out1) -> Degrees to Radians3/1
  Subsystem2/1(Out1) -> Degrees to Radians2/1
  Radians to Degrees2/1 -> Subsystem2/1(In1)
  Demux/1 -> Cartesian to Spherical/1
  Demux/2 -> Cartesian to Spherical/2
  Demux/3 -> Cartesian to Spherical/3
  Mux/1 -> Zero-Order Hold1/1
  Cartesian to Spherical/1 -> Spherical to Cartesian/1
  Spherical to Cartesian/3 -> Mux/3
  Spherical to Cartesian/2 -> Mux/2
  Spherical to Cartesian/1 -> Mux/1
  Cartesian to Spherical/2 -> Radians to Degrees2/1
  Degrees to Radians2/1 -> Spherical to Cartesian/2
  Cartesian to Spherical/3 -> Radians to Degrees3/1
  Degrees to Radians3/1 -> Spherical to Cartesian/3
  Matrix Multiply1/1 -> Demux/1
  Sun position - Body frame/1 -> Matrix Multiply1/2
  Zero-Order Hold1/1 -> [SunSensor_s_B]
  [SunSensor_s_B] -> Scope/1, SunSensor_s_B/1, To Workspace/1
